simulink model "BackEMF_Sensor"  (R2019b)
settings: Solver=VariableStepAuto  StartTime=0.0  StopTime=10.0  RelTol=1e-3
PreLoadFcn:
  | modelDir = fileparts(get_param(bdroot, 'FileName'));
  | addpath(fullfile(modelDir,'../../Parameters'));
  | 
  | Parameters_Model
  | Parameters_Simulation
  | Parameters_Estimators
InitFcn:
  | Parameters_Model
  | Parameters_Simulation
  | Parameters_Estimators
undefined symbols (not defined in the file): ADC_Resolution, ADC_Vref, BackEMF_BAT30_ForwardVoltage, BackEMF_BigRange_VoltageDivider, EnableADCquantization, EnableNoise, sensor_sigma2_backemf, Ts_backemf
settings Model: Creator=Thomas  LastModifiedBy=thomas.jespersen
settings DataIOCC: ReturnWorkspaceOutputs=off
settings DebuggingCC: ArithmeticOperatorsInVariantConditions=warning
settings SFSimCC: SimUseLocalCustomCode=off  CustomCodeUndefinedFunction=UseInterfaceOnly
settings RTWCC: RTWUseLocalCustomCode=off

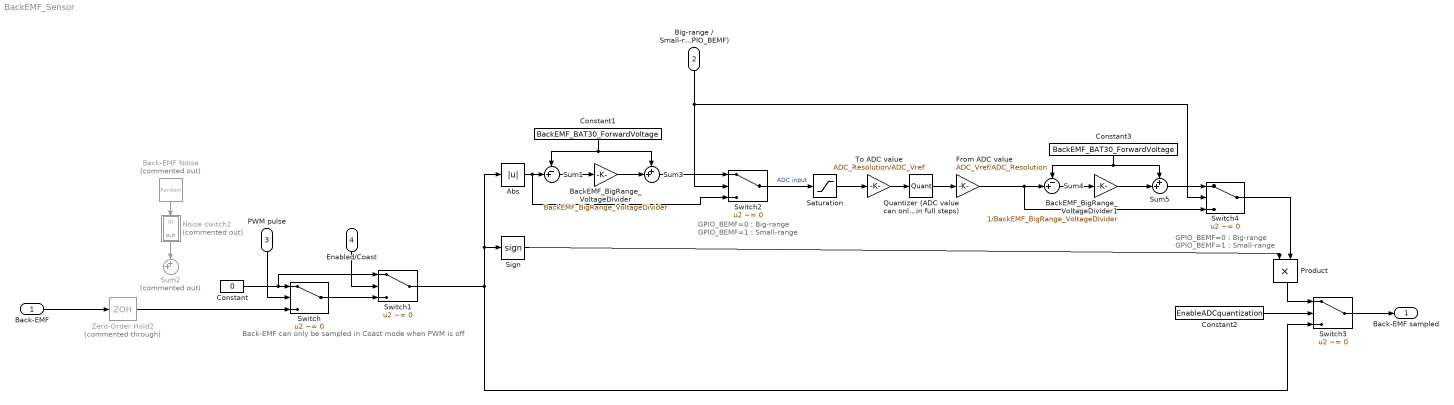
== system BackEMF_Sensor ==
  note: GPIO_BEMF=0 : Big-range
      | GPIO_BEMF=1 : Small-range
  note: Back-EMF can only be sampled in Coast mode when PWM is off
  note: GPIO_BEMF=0 : Big-range
      | GPIO_BEMF=1 : Small-range
  Back-EMF : Inport
  Big-range / Small-range  (GPIO_BEMF) : Inport  Port=2  OutDataTypeStr=boolean
  PWM pulse : Inport  Port=3  OutDataTypeStr=int8
  Enabled/Coast : Inport  Port=4  OutDataTypeStr=boolean
  Abs : Abs
  Back-EMF Noise : RandomNumber  Commented=on  Variance=sensor_sigma2_backemf  Seed=42  SampleTime=Ts_backemf
  BackEMF_BigRange_VoltageDivider : Gain  Gain=BackEMF_BigRange_VoltageDivider
  BackEMF_BigRange_VoltageDivider1 : Gain  Gain=1/BackEMF_BigRange_VoltageDivider
  Constant : Constant  Value=0
  Constant1 : Constant  Value=BackEMF_BAT30_ForwardVoltage
  Constant2 : Constant  Value=EnableADCquantization
  Constant3 : Constant  Value=BackEMF_BAT30_ForwardVoltage
  From ADC value : Gain  Gain=ADC_Vref/ADC_Resolution
  Noise switch2 : Subsystem  Commented=on
  Product : Product
  Quantizer (ADC value can only be measured in full steps) : Quantizer  QuantizationInterval=1
  Saturation : Saturate  UpperLimit=ADC_Vref  LowerLimit=0
  Sign : Signum
  Sum1 : Sum  Inputs=-+|
  Sum2 : Sum  Commented=on  Inputs=++|
  Sum3 : Sum  Inputs=++|
  Sum4 : Sum  Inputs=-+|
  Sum5 : Sum  Inputs=++|
  Switch{,1..4} (5 alike) : Switch  Criteria=u2 ~= 0
  To ADC value : Gain  Gain=ADC_Resolution/ADC_Vref
  Zero-Order Hold2 : ZeroOrderHold  Commented=through  SampleTime=Ts_backemf
  Back-EMF sampled : Outport  VectorParamsAs1DForOutWhenUnconnected=off
  wires:
  Big-range / Small-range  (GPIO_BEMF)/1 -> Switch4/2, Switch2/2
  Constant1/1 -> Sum1/1, Sum3/1
  Sum1/1 -> BackEMF_BigRange_VoltageDivider/1
  Constant/1 -> Switch1/1, Switch/1
  Enabled/Coast/1 -> Switch1/2
  Switch/1 -> Switch1/3
  PWM pulse/1 -> Switch/2
  Zero-Order Hold2/1 -> Switch/3
  Switch3/1 -> Back-EMF sampled/1
  Constant2/1 -> Switch3/2
  To ADC value/1 -> Quantizer (ADC value can only be measured in full steps)/1
  Quantizer (ADC value can only be measured in full steps)/1 -> From ADC value/1
  Switch1/1 -> Sign/1, Abs/1, Switch3/3
  Switch2/1 -> Saturation/1  "ADC input"
  From ADC value/1 -> Sum4/2, Switch4/3
  BackEMF_BigRange_VoltageDivider/1 -> Sum3/2
  Sum3/1 -> Switch2/1
  Sum4/1 -> BackEMF_BigRange_VoltageDivider1/1
  Constant3/1 -> Sum5/1, Sum4/1
  BackEMF_BigRange_VoltageDivider1/1 -> Sum5/2
  Sum5/1 -> Switch4/1
  Switch4/1 -> Product/2
  Abs/1 -> Switch2/3, Sum1/2
  Product/1 -> Switch3/1
  Sign/1 -> Product/1
  Back-EMF/1 -> Zero-Order Hold2/1
  Saturation/1 -> To ADC value/1
  Noise switch2/1(out) -> Sum2/1
  Back-EMF Noise/1 -> Noise switch2/1(in)

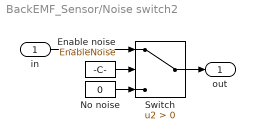
== system BackEMF_Sensor/Noise switch2 ==
  in : Inport
  Enable noise : Constant  Value=EnableNoise
  No noise : Constant  Value=0
  Switch : Switch  Criteria=u2 > Threshold
  out : Outport  VectorParamsAs1DForOutWhenUnconnected=off
  wires:
  No noise/1 -> Switch/3
  Switch/1 -> out/1
  Enable noise/1 -> Switch/2
  in/1 -> Switch/1
